simulink model "Junior_Project_Sim"  (R2016b)
settings: Solver=VariableStepAuto  StartTime=0.0  StopTime=10.0  RelTol=1e-3
values from neighbouring files (symbols this model uses):
  q = 1/2*(rho)*(v)^2    (= 1762.97253125)    [sim_init_junior_project.m]
libraries: simulink x2
settings Model: Creator=Ryan  LastModifiedBy=Ryan

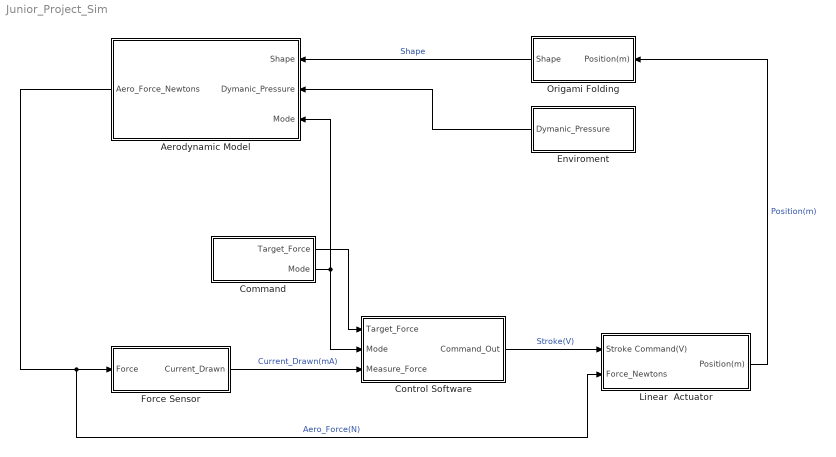
== system Junior_Project_Sim ==
  "  Enviroment" : Subsystem
  " Command" : Subsystem
  " Origami Folding" : Subsystem
  Aerodynamic Model : Subsystem
  Control Software : Subsystem
  Force Sensor : Subsystem
  Linear  Actuator : Subsystem
  wires:
  Control Software/1(Command_Out) -> Linear  Actuator/1(Stroke Command(V))  "Stroke(V)"
  Force Sensor/1(Current_Drawn) -> Control Software/3(Measure_Force)  "Current_Drawn(mA)"
  Aerodynamic Model/1(Aero_Force_Newtons) -> Linear  Actuator/2(Force_Newtons), Force Sensor/1(Force)  "Aero_Force(N)"
  Linear  Actuator/1(Position(m)) -> " Origami Folding"/1(Position(m))  "Position(m)"
  " Origami Folding"/1(Shape) -> Aerodynamic Model/1(Shape)  "Shape"
  " Command"/1(Target_Force) -> Control Software/1(Target_Force)
  "  Enviroment"/1(Dymanic_Pressure) -> Aerodynamic Model/2(Dymanic_Pressure)
  " Command"/2(Mode) -> Aerodynamic Model/3(Mode), Control Software/2(Mode)

== system Junior_Project_Sim/  Enviroment ==
  q : Constant  Value=q
  Dymanic_Pressure : Outport
  wires:
  q/1 -> Dymanic_Pressure/1

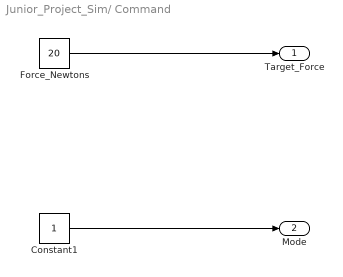
== system Junior_Project_Sim/ Command ==
  Constant1 : Constant
  Force_Newtons : Constant  Value=20
  Target_Force : Outport
  Mode : Outport  Port=2
  wires:
  Force_Newtons/1 -> Target_Force/1
  Constant1/1 -> Mode/1

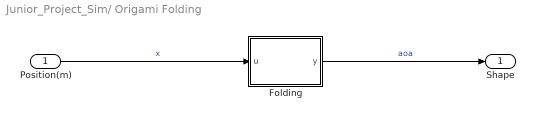
== system Junior_Project_Sim/ Origami Folding ==
  Position(m) : Inport
  Folding : MATLAB Function  TreatAsAtomicUnit=on
  Shape : Outport
  wires:
  Position(m)/1 -> Folding/1(u)  "x"
  Folding/1(y) -> Shape/1  "aoa"

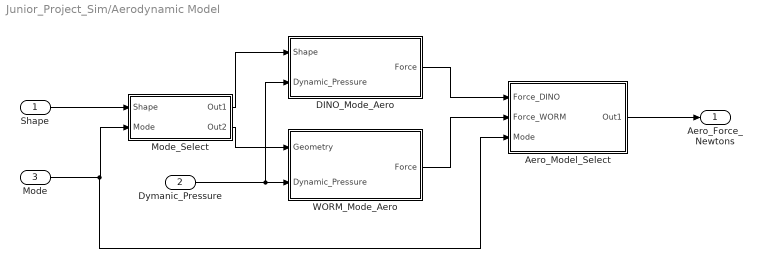
== system Junior_Project_Sim/Aerodynamic Model ==
  Shape : Inport
  Dymanic_Pressure : Inport  Port=2
  Mode : Inport  Port=3
  Aero_Model_Select : Subsystem
  DINO_Mode_Aero : Subsystem
  Mode_Select : Subsystem
  WORM_Mode_Aero : Subsystem
  Aero_Force_Newtons : Outport
  wires:
  Mode_Select/1(Out1) -> DINO_Mode_Aero/1(Shape)
  Mode_Select/2(Out2) -> WORM_Mode_Aero/1(Geometry)
  WORM_Mode_Aero/1(Force) -> Aero_Model_Select/2(Force_WORM)
  DINO_Mode_Aero/1(Force) -> Aero_Model_Select/1(Force_DINO)
  Aero_Model_Select/1(Out1) -> Aero_Force_Newtons/1
  Shape/1 -> Mode_Select/1(Shape)
  Mode/1 -> Aero_Model_Select/3(Mode), Mode_Select/2(Mode)
  Dymanic_Pressure/1 -> DINO_Mode_Aero/2(Dynamic_Pressure), WORM_Mode_Aero/2(Dynamic_Pressure)

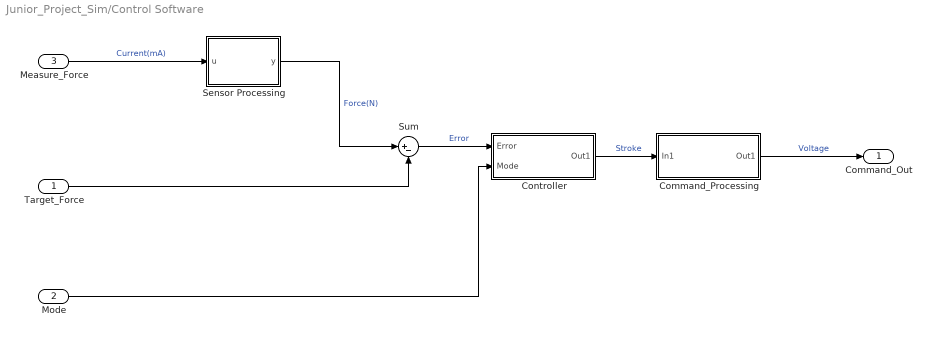
== system Junior_Project_Sim/Control Software ==
  Target_Force : Inport
  Mode : Inport  Port=2
  Measure_Force : Inport  Port=3
  Command_Processing : Subsystem
  Controller : Subsystem
  Sensor Processing : MATLAB Function  TreatAsAtomicUnit=on
  Sum : Sum  Inputs=|+-
  Command_Out : Outport
  wires:
  Measure_Force/1 -> Sensor Processing/1(u)  "Current(mA)"
  Sensor Processing/1(y) -> Sum/1  "Force(N)"
  Command_Processing/1(Out1) -> Command_Out/1  "Voltage"
  Target_Force/1 -> Sum/2
  Controller/1(Out1) -> Command_Processing/1(In1)  "Stroke"
  Sum/1 -> Controller/1(Error)  "Error"
  Mode/1 -> Controller/2(Mode)

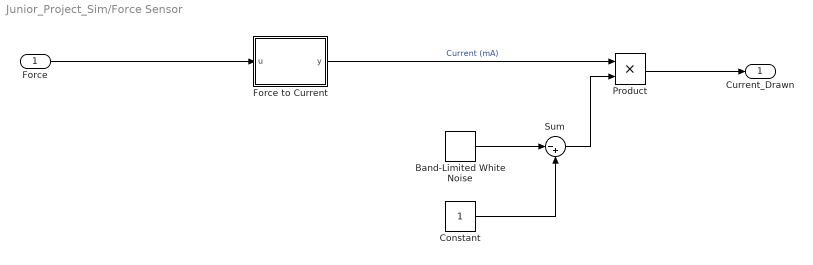
== system Junior_Project_Sim/Force Sensor ==
  Force : Inport
  Band-Limited White Noise : simulink/Sources/Band-Limited White Noise  Cov=[0.01]  Ts=0.1  seed=[23341]
  Constant : Constant
  Force to Current : MATLAB Function  TreatAsAtomicUnit=on
  Product : Product
  Sum : Sum  Inputs=|-+
  Current_Drawn : Outport
  wires:
  Force to Current/1(y) -> Product/1  "Current (mA)"
  Force/1 -> Force to Current/1(u)
  Band-Limited White Noise/1 -> Sum/1
  Product/1 -> Current_Drawn/1
  Constant/1 -> Sum/2
  Sum/1 -> Product/2

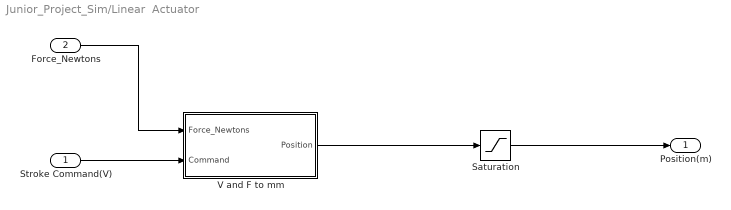
== system Junior_Project_Sim/Linear  Actuator ==
  Stroke Command(V) : Inport
  Force_Newtons : Inport  Port=2
  Saturation : Saturate  UpperLimit=0.140  LowerLimit=0
  V and F to mm : Subsystem
  Position(m) : Outport
  wires:
  Stroke Command(V)/1 -> V and F to mm/2(Command)
  V and F to mm/1(Position) -> Saturation/1
  Force_Newtons/1 -> V and F to mm/1(Force_Newtons)
  Saturation/1 -> Position(m)/1

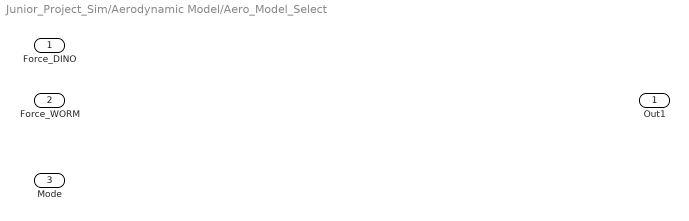
== system Junior_Project_Sim/Aerodynamic Model/Aero_Model_Select ==
  Force_DINO : Inport
  Force_WORM : Inport  Port=2
  Mode : Inport  Port=3
  Out1 : Outport

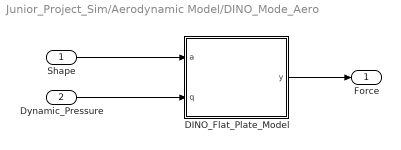
== system Junior_Project_Sim/Aerodynamic Model/DINO_Mode_Aero ==
  Shape : Inport
  Dynamic_Pressure : Inport  Port=2
  DINO_Flat_Plate_Model : MATLAB Function  TreatAsAtomicUnit=on
  Force : Outport
  wires:
  Shape/1 -> DINO_Flat_Plate_Model/1(a)
  Dynamic_Pressure/1 -> DINO_Flat_Plate_Model/2(q)
  DINO_Flat_Plate_Model/1(y) -> Force/1

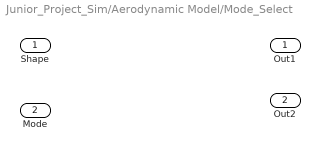
== system Junior_Project_Sim/Aerodynamic Model/Mode_Select ==
  Shape : Inport
  Mode : Inport  Port=2
  Out1 : Outport
  Out2 : Outport  Port=2

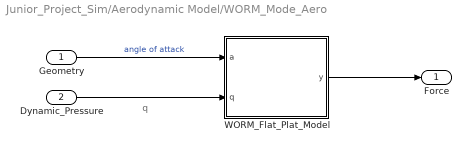
== system Junior_Project_Sim/Aerodynamic Model/WORM_Mode_Aero ==
  note: q
  Geometry : Inport
  Dynamic_Pressure : Inport  Port=2
  WORM_Flat_Plat_Model : MATLAB Function  TreatAsAtomicUnit=on
  Force : Outport
  wires:
  Geometry/1 -> WORM_Flat_Plat_Model/1(a)  "angle of attack"
  WORM_Flat_Plat_Model/1(y) -> Force/1
  Dynamic_Pressure/1 -> WORM_Flat_Plat_Model/2(q)

== system Junior_Project_Sim/Control Software/Command_Processing ==
  In1 : Inport
  Out1 : Outport
  wires:
  In1/1 -> Out1/1

== system Junior_Project_Sim/Control Software/Controller ==
  Error : Inport
  Mode : Inport  Port=2
  Out1 : Outport
  wires:
  Error/1 -> ?

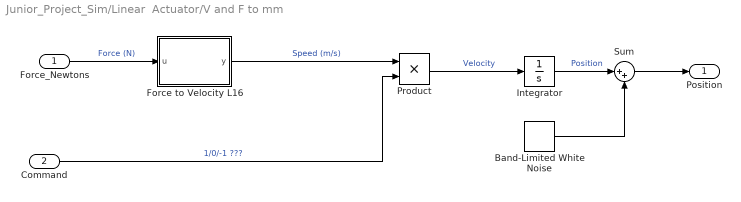
== system Junior_Project_Sim/Linear  Actuator/V and F to mm ==
  Force_Newtons : Inport
  Command : Inport  Port=2
  Band-Limited White Noise : simulink/Sources/Band-Limited White Noise  Cov=0.0003  Ts=0.1  seed=[23342]
  Force to Velocity L16 : MATLAB Function  TreatAsAtomicUnit=on
  Integrator : Integrator
  Product : Product
  Sum : Sum  Inputs=|++
  Position : Outport
  wires:
  Product/1 -> Integrator/1  "Velocity"
  Integrator/1 -> Sum/1  "Position"
  Command/1 -> Product/2  "1/0/-1 ???"
  Force_Newtons/1 -> Force to Velocity L16/1(u)  "Force (N)"
  Force to Velocity L16/1(y) -> Product/1  "Speed (m/s)"
  Band-Limited White Noise/1 -> Sum/2
  Sum/1 -> Position/1

== matlab function Junior_Project_Sim/Aerodynamic Model/WORM_Mode_Aero/WORM_Flat_Plat_Model ==
  data: a input; y output; q input
function y = fcn(a,q)

CD_Plate = -0.9*cos(2*a) + 0.9;

y = CD_Plate.*q*FrontPlateLength*Width;

== matlab function Junior_Project_Sim/Linear  Actuator/V and F to mm/Force to Velocity L16 ==
  data: u input; y output
function y = fcn(u)


y = (-(4/200).*u + 8)*1000;

== matlab function Junior_Project_Sim/Aerodynamic Model/DINO_Mode_Aero/DINO_Flat_Plate_Model ==
  data: a input; y output; q input
function y = fcn(a,q)

CD_Plate = -0.9.*cos(2.*a) + 0.9;

y = CD_Plate.*q.*(2.*FrontPlateLength*Width + FrontPlateLength^2/2.*acos((cos(a)).^2));

== matlab function Junior_Project_Sim/Force Sensor/Force to Current ==
  data: u input; y output
function y = fcn(u)

y = ((400-55)/200).*u + 55;

== matlab function Junior_Project_Sim/Control Software/Sensor Processing ==
  data: u input; y output
function y = fcn(u)

y = (u - 55).*(200/345);

== matlab function Junior_Project_Sim/ Origami Folding/Folding ==
  data: u input; y output
function y = fcn(u)

 index = 0;
 e_previous = 100;
for i = 1:length(Ax(:,1))
    e_current = abs(u - Ax(i,1));
    
    if e_current < e_previous
        index = i;
    else
        %do nothing   
    end
    
end
y = Ax(index,2);
